simulink model "IKS02A1_VL53L1A1_Both_ROS_fromworkspace_2025b_forstudents"  (R2025b)
settings: Solver=VariableStepAuto  StartTime=0.0  StopTime=out.GT_time.time(end)  RelTol=1e-3
libraries: quarc_library x2
settings Model: Creator=abich  LastModifiedBy=tmood

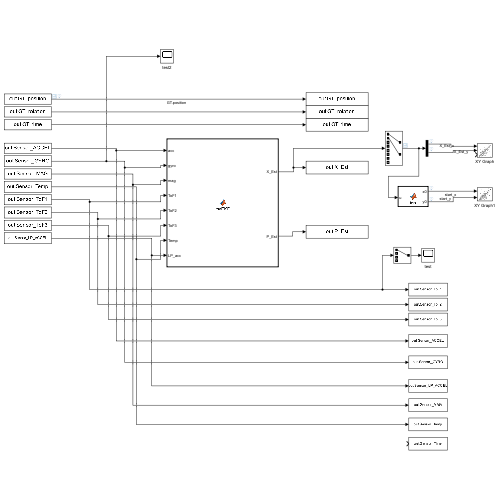
[thumbnail: Simulink's stored preview of the top-level diagram]
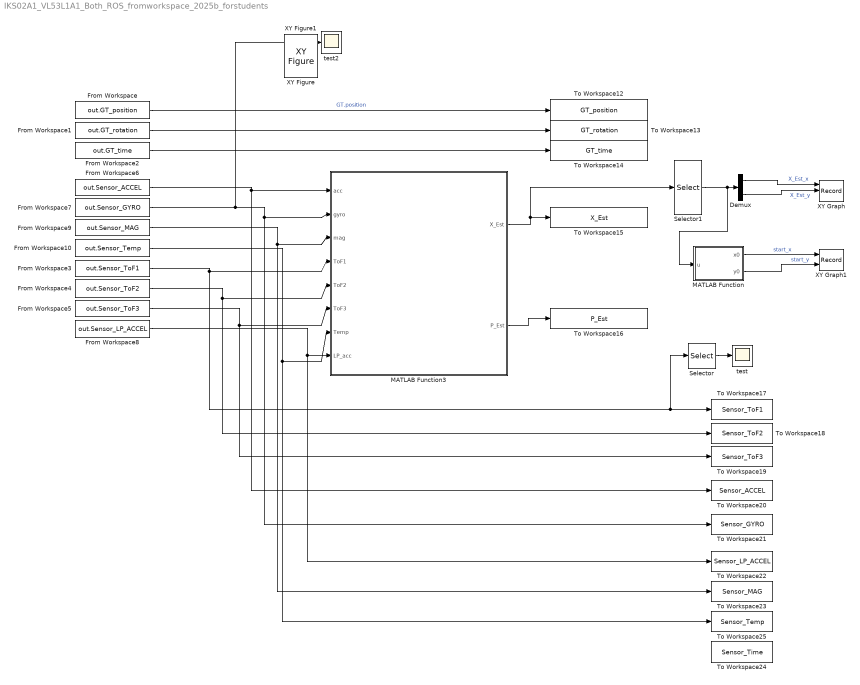
== system IKS02A1_VL53L1A1_Both_ROS_fromworkspace_2025b_forstudents ==
  Demux : Demux  Outputs=2
  From Workspace : FromWorkspace  VariableName=out.GT_position  SampleTime=1/200  OutputAfterFinalValue=Holding final value
  From Workspace1 : FromWorkspace  VariableName=out.GT_rotation  SampleTime=1/200  OutputAfterFinalValue=Holding final value
  From Workspace10 : FromWorkspace  VariableName=out.Sensor_Temp  SampleTime=1/200  OutputAfterFinalValue=Holding final value
  From Workspace2 : FromWorkspace  VariableName=out.GT_time  SampleTime=1/200  OutputAfterFinalValue=Holding final value
  From Workspace3 : FromWorkspace  VariableName=out.Sensor_ToF1  SampleTime=1/200  OutputAfterFinalValue=Holding final value
  From Workspace4 : FromWorkspace  VariableName=out.Sensor_ToF2  SampleTime=1/200  OutputAfterFinalValue=Holding final value
  From Workspace5 : FromWorkspace  VariableName=out.Sensor_ToF3  SampleTime=1/200  OutputAfterFinalValue=Holding final value
  From Workspace6 : FromWorkspace  VariableName=out.Sensor_ACCEL  SampleTime=1/200  OutputAfterFinalValue=Holding final value
  From Workspace7 : FromWorkspace  VariableName=out.Sensor_GYRO  SampleTime=1/200  OutputAfterFinalValue=Holding final value
  From Workspace8 : FromWorkspace  VariableName=out.Sensor_LP_ACCEL  SampleTime=1/200  OutputAfterFinalValue=Holding final value
  From Workspace9 : FromWorkspace  VariableName=out.Sensor_MAG  SampleTime=1/200  OutputAfterFinalValue=Holding final value
  MATLAB Function : MATLAB Function  TreatAsAtomicUnit=on
  MATLAB Function3 : MATLAB Function  TreatAsAtomicUnit=on
  Selector : Selector  InputPortWidth=4  IndexOptions=Index vector (dialog)  Indices=[1]  OutputSizes=1
  Selector1 : Selector  InputPortWidth=8  IndexOptions=Index vector (dialog)  Indices=[1 2]  OutputSizes=1
  To Workspace12 : ToWorkspace  VariableName=GT_position  SaveFormat=Structure With Time  SampleTime=1/200
  To Workspace13 : ToWorkspace  VariableName=GT_rotation  SaveFormat=Structure With Time  SampleTime=1/200
  To Workspace14 : ToWorkspace  VariableName=GT_time  SaveFormat=Structure With Time  SampleTime=1/200
  To Workspace15 : ToWorkspace  VariableName=X_Est  SaveFormat=Structure With Time  SampleTime=1/200
  To Workspace16 : ToWorkspace  VariableName=P_Est  SaveFormat=Structure With Time  SampleTime=1/200
  To Workspace17 : ToWorkspace  VariableName=Sensor_ToF1  SaveFormat=Structure With Time  SampleTime=1/200
  To Workspace18 : ToWorkspace  VariableName=Sensor_ToF2  SaveFormat=Structure With Time  SampleTime=1/200
  To Workspace19 : ToWorkspace  VariableName=Sensor_ToF3  SaveFormat=Structure With Time  SampleTime=1/200
  To Workspace20 : ToWorkspace  VariableName=Sensor_ACCEL  SaveFormat=Structure With Time  SampleTime=1/200
  To Workspace21 : ToWorkspace  VariableName=Sensor_GYRO  SaveFormat=Structure With Time  SampleTime=1/200
  To Workspace22 : ToWorkspace  VariableName=Sensor_LP_ACCEL  SaveFormat=Structure With Time  SampleTime=1/200
  To Workspace23 : ToWorkspace  VariableName=Sensor_MAG  SaveFormat=Structure With Time  SampleTime=1/200
  To Workspace24 : ToWorkspace  VariableName=Sensor_Time  SaveFormat=Structure With Time  SampleTime=1/200
  To Workspace25 : ToWorkspace  VariableName=Sensor_Temp  SaveFormat=Structure With Time  SampleTime=1/200
  XY Graph : Record  NumPorts=3.0  FileSettingsInternal="{\"entries\":[{\"content\":{\"excelSettings\":{\"content\":{},\"type\":\"Streamout.ExcelSettings\"},\"parquetSettings\":{\"content\":{},\"type\":\"Streamout.ParquetSettings\"}},\"type\":\"Streamout.FileSettingStorage\",\"uuid\":\"\"}],\"packageUris\":[\"http:\\/\\/schema.mathworks.com\\/mf0\\/streamout_blocks\\/R2020a\"],\"version\":\"1.0\"}"  FrameSettings=[0, 0, 0]  Layout=[1 1]  SignalsInternal="{\"entries\":[{\"content\":{\"signals\":[{\"content\":{\"blockPath\":[],\"dimensions\":[1],\"domain\":\"\",\"lineColor\":\"#a2142f\",\"plots\":[ 1 ],\"port\":1,\"sid\":[\"\"],\"signalID\":1,\"signalName\":\"X_Est_x\"},\"type\":\"RecordBlkView.Signal\",\"uuid\":\"\"},{\"content\":{\"blockPath\":[],\"dimensions\":[1],\"domain\":\"\",\"lineColor\":\"#139fff\",\"plots\":[ 1 ],\"port\":2,\"sid\":[\"\"],\"signalID\":2,\"signalName\":\"X_Est_y\"},\"type\":\"RecordBlkView.Signal\",\"uuid\":\"\"},{\"content\":{\"blockPath\":[],\"dimensions\":[1],\"domain\":\"\",\"lineColor\":\"#139fff\",\"lineWidth\":2,\"port\":3,\"sid\":[\"\"],\"signalID\":3},\"type\":\"RecordBlkView.Signal\",\"uuid\":\"\"}]},\"type\":\"RecordBlkView.InputSignals\",\"uuid\":\"\"}],\"packageUris\":[\"http:\\/\\/schema.mathworks.com\\/mf0\\/streamout_blocks\\/R2020a\"],\"version\":\"1.0\"}"  VisualizationBindings="{\"xyplotplugin\":{\"info\":[{\"series\":[{\"bindingParametersList\":[{\"parameter\":\"X-Axis\",\"signalID\":1,\"signalName\":\"X_Est_x\"},{\"parameter\":\"Y-Axis\",\"signalID\":2,\"signalName\":\"X_Est_y\"}],\"seriesID\":0}],\"subplotID\":1}]}}"  CompatibilityTag=XY
  XY Graph1 : Record  NumPorts=2.0  FileSettingsInternal="{\"entries\":[{\"content\":{\"excelSettings\":{\"content\":{},\"type\":\"Streamout.ExcelSettings\"},\"parquetSettings\":{\"content\":{},\"type\":\"Streamout.ParquetSettings\"}},\"type\":\"Streamout.FileSettingStorage\",\"uuid\":\"\"}],\"packageUris\":[\"http:\\/\\/schema.mathworks.com\\/mf0\\/streamout_blocks\\/R2020a\"],\"version\":\"1.0\"}"  FrameSettings=[0, 0]  Layout=[1 1]  SignalsInternal="{\"entries\":[{\"content\":{\"signals\":[{\"content\":{\"blockPath\":[],\"dimensions\":[1],\"domain\":\"\",\"lineColor\":\"#a2142f\",\"plots\":[ 1 ],\"port\":1,\"sid\":[\"\"],\"signalID\":1,\"signalName\":\"start_x\"},\"type\":\"RecordBlkView.Signal\",\"uuid\":\"\"},{\"content\":{\"blockPath\":[],\"dimensions\":[1],\"domain\":\"\",\"lineColor\":\"#139fff\",\"plots\":[ 1 ],\"port\":2,\"sid\":[\"\"],\"signalID\":2,\"signalName\":\"start_y\"},\"type\":\"RecordBlkView.Signal\",\"uuid\":\"\"}]},\"type\":\"RecordBlkView.InputSignals\",\"uuid\":\"\"}],\"packageUris\":[\"http:\\/\\/schema.mathworks.com\\/mf0\\/streamout_blocks\\/R2020a\"],\"version\":\"1.0\"}"  VisualizationBindings="{\"xyplotplugin\":{\"info\":[{\"series\":[{\"bindingParametersList\":[{\"parameter\":\"X-Axis\",\"signalID\":1,\"signalName\":\"start_x\"},{\"parameter\":\"Y-Axis\",\"signalID\":2,\"signalName\":\"start_y\"}],\"seriesID\":0}],\"subplotID\":1}]}}"  CompatibilityTag=XY
  test : Scope
      settings: ActiveDisplayYMinimum=-1  ActiveDisplayYMaximum=1
  test2 : Scope
      settings: ActiveDisplayYMinimum=-0.15108420974985681  ActiveDisplayYMaximum=0.16772460685752888  DataLoggingVariableName=ScopeData2
  XY Figure : quarc_library/Sinks/Figures/XY Figure  IOType=viewer  figure_mode=Use figure window  figure_tag=figure1  axes_tag=axes1  plot_mode=Time-based  minimum_x=-1  maximum_x=1  minimum_y=-1  maximum_y=1  buffer_size=1000  update_rate=100  initial_position=[]  initial_visibility=off  sample_time=-1
      settings: SourceProductName=QUARC Targets
  XY Figure1 : quarc_library/Sinks/Figures/XY Figure  IOType=viewer  figure_mode=Use figure window  figure_tag=figure1  axes_tag=axes1  plot_mode=Time-based  minimum_x=-1  maximum_x=1  minimum_y=-1  maximum_y=1  buffer_size=1000  update_rate=100  initial_position=[]  initial_visibility=off  sample_time=-1
      settings: SourceProductName=QUARC Targets
  wires:
  From Workspace4/1 -> To Workspace18/1, MATLAB Function3/5(ToF2)
  From Workspace6/1 -> To Workspace20/1, MATLAB Function3/1(acc)
  From Workspace9/1 -> To Workspace23/1, MATLAB Function3/3(mag)
  From Workspace10/1 -> To Workspace25/1, MATLAB Function3/7(Temp)
  From Workspace2/1 -> To Workspace14/1
  From Workspace5/1 -> To Workspace19/1, MATLAB Function3/6(ToF3)
  MATLAB Function3/1(X_Est) -> Selector1/1, To Workspace15/1
  From Workspace8/1 -> MATLAB Function3/8(LP_acc), To Workspace22/1
  From Workspace3/1 -> Selector/1, To Workspace17/1, MATLAB Function3/4(ToF1)
  From Workspace1/1 -> To Workspace13/1
  From Workspace7/1 -> test2/1, To Workspace21/1, MATLAB Function3/2(gyro)
  MATLAB Function3/2(P_Est) -> To Workspace16/1
  Selector/1 -> test/1
  Selector1/1 -> MATLAB Function/1(u), Demux/1
  Demux/1 -> XY Graph/1  "X_Est_x"
  Demux/2 -> XY Graph/2  "X_Est_y"
  From Workspace/1 -> To Workspace12/1  "GT.position"
  MATLAB Function/1(x0) -> XY Graph1/1  "start_x"
  MATLAB Function/2(y0) -> XY Graph1/2  "start_y"

== matlab function IKS02A1_VL53L1A1_Both_ROS_fromworkspace_2025b_forstudents/MATLAB Function ==
  data: u input; x0 output; y0 output
function [x0,y0] = fcn(u)

x0 = u(1,1);
y0 = u(2,1);
end

== matlab function IKS02A1_VL53L1A1_Both_ROS_fromworkspace_2025b_forstudents/MATLAB Function3 ==
  data: acc input; X_Est output size=8; gyro input; mag input; ToF1 input; ToF2 input; ToF3 input; P_Est output size=[5 5]; Temp input; LP_acc input
function [X_Est, P_Est] = myEKF(acc, gyro, mag, ToF1, ToF2, ToF3, Temp, LP_acc)
% EKF for Sub-Terranean Navigation — Simulink MATLAB Function Block
% Called once per timestep (200Hz, dt=0.005s)
% Inputs (per timestep):
%   acc    : 3x1 accelerometer [ax; ay; az] m/s²
%   gyro   : 3x1 gyroscope     [gx; gy; gz] rad/s  (gx = yaw axis)
%   mag    : 3x1 magnetometer  [mx; my; mz] Tesla
%   ToF1   : 4x1 [dist; ?; ?; status]  left-facing   (alpha=+pi/2)    % *** CHANGED: was right
%   ToF2   : 4x1 [dist; ?; ?; status]  back-facing   (alpha=pi)       % *** CHANGED: was forward
%   ToF3   : 4x1 [dist; ?; ?; status]  right-facing  (alpha=-pi/2)    % *** CHANGED: was left
%   Temp   : unused (template placeholder)
%   LP_acc : unused (template placeholder)
% Outputs:
%   X_Est  : 1x5 [x, y, theta, vx_world, vy_world]
%   P_Est  : 5x5 covariance (top-left block)

%% Persistent state — survives between Simulink timestep calls
persistent X P initialized call_count

% Calibration (computed during startup)
persistent gyro_bias accel_bias_fwd accel_bias_lat
persistent x0 y0 mag_global_offset
persistent ab_xmax ab_xmin ab_ymax ab_ymin

% Mag anomaly detection
persistent theta_gyro_ref gyro_ref_bias mag_disable_until
persistent mag_innov_buf mag_innov_count
persistent gyro_mag_diverge_count prev_innovation_mag mag_innov_growing_count

% ToF rate tracking
persistent prev_tof1_dist prev_tof1_genuine_time
persistent prev_tof2_dist prev_tof2_genuine_time
persistent prev_tof3_dist prev_tof3_genuine_time

% Startup accumulation buffers
persistent startup_gyro startup_accel startup_tof1 startup_tof2 startup_tof3
persistent startup_mag startup_done startup_buf_count

persistent zupt_accel_fwd_buf zupt_accel_lat_buf zupt_gyro_buf zupt_buf_count

%% Constants
dt              = 0.005;

% *** CHANGED: Corrected ToF mounting angles (confirmed by diagnostic) ***
alpha_tof1      =  pi/2;   % was -pi/2 — ToF1 = left
alpha_tof2      =  pi;     % was  0    — ToF2 = back
alpha_tof3      = -pi/2;   % was  pi/2 — ToF3 = right

mag_hard_iron   = [-3.705e-05,  4.415e-05];
mag_soft_iron   = [ 1.0958,     0.9196   ];
theta0          = pi/2;
R_mag           = 4.0;
R_tof           = 0.01;
gamma_threshold = 9.0;

%% First call: initialise all persistent variables
if isempty(initialized)
    call_count   = 0;
    startup_done = false;
    startup_buf_count = 0;

    % Startup buffers — pre-allocate for up to 500 samples
    startup_gyro  = zeros(500, 3);
    startup_accel = zeros(500, 3);
    startup_tof1  = zeros(500, 4);
    startup_tof2  = zeros(500, 4);
    startup_tof3  = zeros(500, 4);
    startup_mag   = zeros(500, 3);

    % Fallback calibration constants (used if startup fails)
    gyro_bias      =  0.00186;
    accel_bias_fwd = -0.396;
    accel_bias_lat =  0.07485;
    x0             =  0.0;
    y0             = -0.93;

    % ZUPT
    zupt_accel_fwd_buf = zeros(40, 1);
    zupt_accel_lat_buf = zeros(40, 1);
    zupt_gyro_buf      = zeros(40, 1);
    zupt_buf_count     = 0;

    % arena_bounds = struct('x_max',  1.22, 'x_min', -1.22, ...
    %                       'y_max',  1.22, 'y_min', -1.22);
    ab_xmax =  1.22; ab_xmin = -1.22;
    ab_ymax =  1.22; ab_ymin = -1.22;

    % These will be properly set after startup completes
    mag_global_offset       = 0;
    theta_gyro_ref          = theta0;
    gyro_ref_bias           = gyro_bias;
    mag_disable_until       = 0;
    mag_innov_buf           = zeros(20, 1);
    mag_innov_count         = 0;
    gyro_mag_diverge_count  = 0;
    prev_innovation_mag     = 0;
    mag_innov_growing_count = 0;

    prev_tof1_dist         = NaN;
    prev_tof1_genuine_time = NaN;
    prev_tof2_dist         = NaN;
    prev_tof2_genuine_time = NaN;
    prev_tof3_dist         = NaN;
    prev_tof3_genuine_time = NaN;

    % State and covariance — will be reset after startup
    X = [0; -0.93; theta0; 0; 0; gyro_bias];
    P = diag([0.1, 0.1, 0.1, 2.0, 2.0, 0.25]);

    initialized = true;
end

call_count = call_count + 1;
current_time = (call_count - 1) * dt;

%% Startup phase: accumulate samples, compute calibration
if ~startup_done
    startup_buf_count = startup_buf_count + 1;
    n = min(startup_buf_count, 500);
    startup_gyro(n, :)  = reshape(gyro,  1, 3);
    startup_accel(n, :) = reshape(acc,   1, 3);
    startup_mag(n, :)   = reshape(mag,   1, 3);
    startup_tof1(n, :)  = reshape(ToF1,  1, 4);
    startup_tof2(n, :)  = reshape(ToF2,  1, 4);
    startup_tof3(n, :)  = reshape(ToF3,  1, 4);

    % *** CHANGED: Use variance-based stationarity detection instead of ***
    % *** absolute threshold. The gyro has a large bias (~-0.49 rad/s)  ***
    % *** so abs(gyro(1)) < 0.01 never triggers. Instead, check if the ***
    % *** gyro reading is STABLE (low variance) over a window.          ***
    if startup_buf_count >= 100
        stat_start   = 0;
        search_limit = min(startup_buf_count, 500);

        % Look for a window of 100 samples where gyro variance is low
        % (robot stationary = constant gyro reading = low variance)
        for i = 100:search_limit
            window = startup_gyro((i-99):i, 1);
            win_var = var(window);
            if win_var < 1e-4   % Low variance = stationary, regardless of bias value
                stat_start = i - 99;
                break;
            end
        end

        if stat_start > 0
            n_stat     = min(200, search_limit - stat_start + 1);
            stat_range = stat_start : (stat_start + n_stat - 1);

            % Per-run calibration
            gyro_bias      = mean(startup_gyro(stat_range, 1));
            accel_bias_fwd = mean(startup_accel(stat_range, 3));
            accel_bias_lat = mean(startup_accel(stat_range, 2));

            % Arena wall + x0/y0 estimation from ToF
            tof1_in = startup_tof1(stat_range, 1);
            tof2_in = startup_tof2(stat_range, 1);
            tof3_in = startup_tof3(stat_range, 1);

            gen1 = tof1_in([true; diff(tof1_in) ~= 0]);
            gen2 = tof2_in([true; diff(tof2_in) ~= 0]);
            gen3 = tof3_in([true; diff(tof3_in) ~= 0]);
            gen1 = gen1(gen1 > 0);
            gen2 = gen2(gen2 > 0);
            gen3 = gen3(gen3 > 0);

            if ~isempty(gen1) && ~isempty(gen2) && ~isempty(gen3)
                s1 = sort(gen1); d_lft = s1(max(1,floor(end/2)));  % *** CHANGED: ToF1=left (was d_rgt)
                s2 = sort(gen2); d_bck = s2(max(1,floor(end/2)));  % *** CHANGED: ToF2=back (was d_fwd)
                s3 = sort(gen3); d_rgt = s3(max(1,floor(end/2)));  % *** CHANGED: ToF3=right (was d_lft)

                if d_lft > 0 && d_bck > 0 && d_rgt > 0 && ...
                   ~isnan(d_lft) && ~isnan(d_bck) && ~isnan(d_rgt)

                    % *** CHANGED: Position estimation using correct ToF mapping ***
                    % At theta0=pi/2: left(+pi/2)=back(+Y), back(pi)=right(+X), right(-pi/2)=forward(-Y)
                    % Actually at theta=pi/2:
                    %   ToF1 left  (+pi/2 from heading): ray = pi/2+pi/2 = pi   → points -X direction → measures dist to -X wall
                    %   ToF2 back  (pi from heading):    ray = pi/2+pi = 3pi/2  → points -Y direction → measures dist to -Y wall
                    %   ToF3 right (-pi/2 from heading): ray = pi/2-pi/2 = 0    → points +X direction → measures dist to +X wall
                    wall_x_max =  1.22;
                    wall_y_max =  1.22;
                    wall_x_min = -1.22;
                    wall_y_min = -1.22;

                    x0 = wall_x_max - d_rgt;     % d_rgt = dist to +X wall
                    y0 = wall_y_min + d_bck;      % d_bck = dist to -Y wall (behind at theta=pi/2 means -Y)

                    % Verify with left sensor: x0 should be close to wall_x_min + d_lft
                    % x0_check = wall_x_min + d_lft;

                    ab_xmax = wall_x_max;
                    ab_xmin = wall_x_min;
                    ab_ymax = wall_y_max;
                    ab_ymin = wall_y_min;
                end
            end

            % Magnetometer global offset
            % *** CHANGED: Use first valid (non-zero) mag sample ***
            mag_init_idx = 1;
            for mi = 1:min(startup_buf_count, 500)
                if norm(startup_mag(mi,:)) > 1e-8
                    mag_init_idx = mi;
                    break;
                end
            end
            mag_y_cal0        = (startup_mag(mag_init_idx,2) - mag_hard_iron(1)) * mag_soft_iron(1);
            mag_z_cal0        = (startup_mag(mag_init_idx,3) - mag_hard_iron(2)) * mag_soft_iron(2);
            z_mag0            = atan2(mag_z_cal0, mag_y_cal0);
            mag_global_offset = wrapToPi_fn(theta0 - z_mag0);

            % Initialise filter state with estimated x0, y0
            X = [x0; y0; theta0; 0; 0; gyro_bias];
            P = diag([0.1, 0.1, 0.1, 2.0, 2.0, 0.25]);

            theta_gyro_ref = theta0;
            gyro_ref_bias  = gyro_bias;

            startup_done = true;
        end
    end

    % During startup, return zero estimates
    X_Est = [0; -0.93; pi/2; 0; 0; 0; 0; 0];   % 1x8
    P_Est = zeros(5, 5);
    return;
end

%% Extract current sensor values
gx      = gyro(1);          % yaw axis gyro (rad/s)
ax_body_raw = acc(3);       % forward accel (m/s²)
ay_body_raw = acc(2);       % lateral accel (m/s²)

tof1_dist   = ToF1(1);
tof1_status = ToF1(4);
tof2_dist   = ToF2(1);
tof2_status = ToF2(4);
tof3_dist   = ToF3(1);
tof3_status = ToF3(4);

mag_y = mag(2);
mag_z = mag(3);

%% Prediction step
omega   = gx - X(6);
Q_base  = diag([1e-4, 1e-4, 1.1e-3, 0.5, 0.5, 1.5e-5]) * dt;

% *** CHANGED: Increased accel clamp from 2.0 to 3.0 — but accel is very ***
% *** noisy (spikes to ±15 m/s²). Consider reducing further or scaling.  ***
ax_body = max(-3.0, min(3.0, ax_body_raw - accel_bias_fwd));
ay_body = max(-3.0, min(3.0, ay_body_raw - accel_bias_lat));

ax_world = ax_body * cos(X(3)) - ay_body * sin(X(3));
ay_world = ax_body * sin(X(3)) + ay_body * cos(X(3));

vel_damp  = 1.0 - 0.5 * dt;

X_pred    = zeros(6, 1);
X_pred(1) = X(1) + X(4) * dt;
X_pred(2) = X(2) + X(5) * dt;
X_pred(3) = wrapToPi_fn(X(3) + omega * dt);
X_pred(4) = X(4) * vel_damp + ax_world * dt;
X_pred(5) = X(5) * vel_damp + ay_world * dt;
X_pred(6) = X(6);

F       = eye(6);
F(1, 4) = dt;
F(2, 5) = dt;
F(3, 6) = -dt;
F(4, 3) = (-ax_body * sin(X(3)) - ay_body * cos(X(3))) * dt;
F(5, 3) = ( ax_body * cos(X(3)) - ay_body * sin(X(3))) * dt;
F(4, 4) = vel_damp;
F(5, 5) = vel_damp;

% Adaptive Q
Q_k = Q_base;
if abs(omega) > 0.15
    Q_k(3,3) = Q_k(3,3) * (1.0 + 9.0 * (abs(omega) - 0.15));
end
if call_count <= mag_disable_until
    Q_k(4,4) = Q_k(4,4) * 1.5;
    Q_k(5,5) = Q_k(5,5) * 1.5;
end
speed = sqrt(X(4)^2 + X(5)^2);
if speed > 0.05
    Q_k(6,6) = Q_k(6,6) * (1.0 + 5.0 * speed);
end

P_pred = F * P * F' + Q_k;
X      = X_pred;
P      = P_pred;

%% Gyro reference update
theta_gyro_ref = wrapToPi_fn(theta_gyro_ref + (gx - gyro_ref_bias) * dt);

%% Magnetometer update with anomaly detection
mag_y_cal = (mag_y - mag_hard_iron(1)) * mag_soft_iron(1);
mag_z_cal = (mag_z - mag_hard_iron(2)) * mag_soft_iron(2);
z_mag     = wrapToPi_fn(atan2(mag_z_cal, mag_y_cal) + mag_global_offset);

innovation_mag = wrapToPi_fn(z_mag - X(3));

% Criterion 1: innovation buffer
mag_innov_count        = mag_innov_count + 1;
buf_idx                = mod(mag_innov_count - 1, 20) + 1;
mag_innov_buf(buf_idx) = innovation_mag;
if mag_innov_count >= 20
    ib_mean   = sum(mag_innov_buf) / 20;
    innov_var = sum((mag_innov_buf - ib_mean).^2) / 19;
    innov_rms = sqrt(sum(mag_innov_buf.^2) / 20);
    if innov_var > 0.04 || innov_rms > 0.15
        mag_disable_until = call_count + 400;
    end
end

% Criterion 2: innovation growing for 5 consecutive steps
if abs(innovation_mag) > abs(prev_innovation_mag) + 0.02
    mag_innov_growing_count = mag_innov_growing_count + 1;
    if mag_innov_growing_count >= 5
        mag_disable_until       = call_count + 400;
        mag_innov_growing_count = 0;
    end
else
    mag_innov_growing_count = max(0, mag_innov_growing_count - 1);
end
prev_innovation_mag = innovation_mag;

% Criterion 3: sustained divergence from gyro reference
gyro_mag_diff = abs(wrapToPi_fn(z_mag - theta_gyro_ref));
max_expected  = 0.008 * current_time + 0.12;
if gyro_mag_diff > max_expected
    gyro_mag_diverge_count = gyro_mag_diverge_count + 1;
    if gyro_mag_diverge_count >= 50
        mag_disable_until      = call_count + 400;
        gyro_mag_diverge_count = 0;
    end
else
    gyro_mag_diverge_count = max(0, gyro_mag_diverge_count - 1);
end

% Apply mag update only when not disabled
if call_count > mag_disable_until
    R_mag_k = 4.0;
    H_mag = [0 0 1 0 0 0];
    S_mag = H_mag * P * H_mag' + R_mag_k;
    if innovation_mag^2 / S_mag < gamma_threshold
        K_mag = P * H_mag' / S_mag;
        X     = X + K_mag * innovation_mag;
        X(3)  = wrapToPi_fn(X(3));
        IKH   = eye(6) - K_mag * H_mag;
        P     = IKH * P * IKH' + K_mag * R_mag_k * K_mag';
        gyro_ref_bias = 0.95 * gyro_ref_bias + 0.05 * X(6);
    end
end

%% ToF distance + rate updates
% ToF 1
if tof1_status == 0
    [h_x, H_tof] = calc_tof(X, ab_xmax, ab_xmin, ab_ymax, ab_ymin, alpha_tof1);
    S          = H_tof * P * H_tof' + R_tof;
    innovation = tof1_dist - h_x;
    if (innovation^2) / S < gamma_threshold
        K    = P * H_tof' / S;
        X    = X + K * innovation;
        X(3) = wrapToPi_fn(X(3));
        IKH  = eye(6) - K * H_tof;
        P    = IKH * P * IKH' + K * R_tof * K';
    end
    tof1_is_new = isnan(prev_tof1_dist) || (tof1_dist ~= prev_tof1_dist);
    if tof1_is_new && ~isnan(prev_tof1_dist) && call_count <= mag_disable_until
        dt_gen = current_time - prev_tof1_genuine_time;
        if dt_gen > 0.08
            spd = sqrt(X(4)^2 + X(5)^2);
            if spd > 0.05 && abs(omega) < 0.2
                phi        = wrapToPi_fn(X(3) + alpha_tof1);
                dro        = (tof1_dist - prev_tof1_dist) / dt_gen;
                dre        = -(X(4)*cos(phi) + X(5)*sin(phi));
                Hr         = zeros(1,6);
                Hr(3)      = X(4)*sin(phi) - X(5)*cos(phi);
                Hr(4)      = -cos(phi);
                Hr(5)      = -sin(phi);
                Sr         = Hr * P * Hr' + 0.5;
                ir         = dro - dre;
                if ir^2 < 9.0 * Sr
                    Kr   = P * Hr' / Sr;
                    X    = X + Kr * ir;
                    X(3) = wrapToPi_fn(X(3));
                    P    = (eye(6) - Kr * Hr) * P;
                end
            end
        end
    end
    if tof1_is_new
        prev_tof1_dist         = tof1_dist;
        prev_tof1_genuine_time = current_time;
    end
end

% ToF 2
if tof2_status == 0
    [h_x, H_tof] = calc_tof(X, ab_xmax, ab_xmin, ab_ymax, ab_ymin, alpha_tof2);
    S          = H_tof * P * H_tof' + R_tof;
    innovation = tof2_dist - h_x;
    if (innovation^2) / S < gamma_threshold
        K    = P * H_tof' / S;
        X    = X + K * innovation;
        X(3) = wrapToPi_fn(X(3));
        IKH  = eye(6) - K * H_tof;
        P    = IKH * P * IKH' + K * R_tof * K';
    end
    tof2_is_new = isnan(prev_tof2_dist) || (tof2_dist ~= prev_tof2_dist);
    if tof2_is_new && ~isnan(prev_tof2_dist) && call_count <= mag_disable_until
        dt_gen = current_time - prev_tof2_genuine_time;
        if dt_gen > 0.08
            spd = sqrt(X(4)^2 + X(5)^2);
            if spd > 0.05 && abs(omega) < 0.2
                phi        = wrapToPi_fn(X(3) + alpha_tof2);
                dro        = (tof2_dist - prev_tof2_dist) / dt_gen;
                dre        = -(X(4)*cos(phi) + X(5)*sin(phi));
                Hr         = zeros(1,6);
                Hr(3)      = X(4)*sin(phi) - X(5)*cos(phi);
                Hr(4)      = -cos(phi);
                Hr(5)      = -sin(phi);
                Sr         = Hr * P * Hr' + 0.5;
                ir         = dro - dre;
                if ir^2 < 9.0 * Sr
                    Kr   = P * Hr' / Sr;
                    X    = X + Kr * ir;
                    X(3) = wrapToPi_fn(X(3));
                    P    = (eye(6) - Kr * Hr) * P;
                end
            end
        end
    end
    if tof2_is_new
        prev_tof2_dist         = tof2_dist;
        prev_tof2_genuine_time = current_time;
    end
end

% ToF 3
if tof3_status == 0
    [h_x, H_tof] = calc_tof(X, ab_xmax, ab_xmin, ab_ymax, ab_ymin, alpha_tof3);
    S          = H_tof * P * H_tof' + R_tof;
    innovation = tof3_dist - h_x;
    if (innovation^2) / S < gamma_threshold
        K    = P * H_tof' / S;
        X    = X + K * innovation;
        X(3) = wrapToPi_fn(X(3));
        IKH  = eye(6) - K * H_tof;
        P    = IKH * P * IKH' + K * R_tof * K';
    end
    tof3_is_new = isnan(prev_tof3_dist) || (tof3_dist ~= prev_tof3_dist);
    if tof3_is_new && ~isnan(prev_tof3_dist) && call_count <= mag_disable_until
        dt_gen = current_time - prev_tof3_genuine_time;
        if dt_gen > 0.08
            spd = sqrt(X(4)^2 + X(5)^2);
            if spd > 0.05 && abs(omega) < 0.2
                phi        = wrapToPi_fn(X(3) + alpha_tof3);
                dro        = (tof3_dist - prev_tof3_dist) / dt_gen;
                dre        = -(X(4)*cos(phi) + X(5)*sin(phi));
                Hr         = zeros(1,6);
                Hr(3)      = X(4)*sin(phi) - X(5)*cos(phi);
                Hr(4)      = -cos(phi);
                Hr(5)      = -sin(phi);
                Sr         = Hr * P * Hr' + 0.5;
                ir         = dro - dre;
                if ir^2 < 9.0 * Sr
                    Kr   = P * Hr' / Sr;
                    X    = X + Kr * ir;
                    X(3) = wrapToPi_fn(X(3));
                    P    = (eye(6) - Kr * Hr) * P;
                end
            end
        end
    end
    if tof3_is_new
        prev_tof3_dist         = tof3_dist;
        prev_tof3_genuine_time = current_time;
    end
end

%% ZUPT — 40-sample variance window
zupt_buf_count = zupt_buf_count + 1;
buf_i = mod(zupt_buf_count - 1, 40) + 1;
zupt_accel_fwd_buf(buf_i) = ax_body;
zupt_accel_lat_buf(buf_i) = ay_body;
zupt_gyro_buf(buf_i)      = gx;

if zupt_buf_count >= 40
    az_mean  = sum(zupt_accel_fwd_buf) / 40;
    ay_mean  = sum(zupt_accel_lat_buf) / 40;
    gy_mean  = sum(zupt_gyro_buf) / 40;
    az_var   = sum((zupt_accel_fwd_buf - az_mean).^2) / 39;
    ay_var   = sum((zupt_accel_lat_buf - ay_mean).^2) / 39;
    gyro_var = sum((zupt_gyro_buf - gy_mean).^2) / 39;

    if az_var < 0.005 && ay_var < 0.005 && gyro_var < 0.0005
        % Part 1: Velocity ZUPT
        H_v     = [0 0 0 1 0 0; 0 0 0 0 1 0];
        innov_v = -[X(4); X(5)];
        S_v     = H_v * P * H_v' + 0.002 * eye(2);
        K_v     = P * H_v' / S_v;
        X       = X + K_v * innov_v;
        P       = (eye(6) - K_v * H_v) * P;

        % Part 2: Gyro bias ZUPT
        H_b     = [0 0 0 0 0 1];
        innov_b = gx - X(6);
        S_b     = P(6,6) + 0.00005;
        K_b     = P * H_b' / S_b;
        X       = X + K_b * innov_b;
        P       = (eye(6) - K_b * H_b) * P;
        gyro_ref_bias = X(6);

        % Part 3: Soft heading ZUPT
        H_h     = [0 0 1 0 0 0];
        innov_h = -(omega * dt);
        S_h     = H_h * P * H_h' + 0.005;
        K_h     = P * H_h' / S_h;
        X       = X + K_h * innov_h;
        X(3)    = wrapToPi_fn(X(3));
        P       = (eye(6) - K_h * H_h) * P;
    end
end

%% Output current state estimate
X_Est = [X(1:5); 0; 0; 0];    % 1x8 — padded to match model expectation
P_Est = P(1:5, 1:5);           % 5x5

end  % function myEKF

%% Local helper: ToF measurement model
function [h_x, H_tof] = calc_tof(X, xmax, xmin, ymax, ymin, alpha)
    x   = X(1);
    y   = X(2);
    phi = mod(X(3) + alpha + pi, 2*pi) - pi;

    d_right  = inf; d_left = inf; d_top = inf; d_bottom = inf;

    if cos(phi) > 1e-6
        d_right = (xmax - x) / cos(phi);
    elseif cos(phi) < -1e-6
        d_left  = (xmin - x) / cos(phi);
    end
    if sin(phi) > 1e-6
        d_top    = (ymax - y) / sin(phi);
    elseif sin(phi) < -1e-6
        d_bottom = (ymin - y) / sin(phi);
    end

    distances = [d_right, d_left, d_top, d_bottom];
    distances(distances <= 0) = inf;
    [h_x, wall_idx] = min(distances);

    if isinf(h_x)
        H_tof = zeros(1, length(X));
        return;
    end

    H_tof = zeros(1, 6);
    if wall_idx == 1 || wall_idx == 2
        H_tof(1) = -1 / cos(phi);
        H_tof(3) = 0;
    else
        H_tof(2) = -1 / sin(phi);
        H_tof(3) = 0;
    end
end

%% Local helper: angle wrapping
function a = wrapToPi_fn(a)
    a = mod(a + pi, 2*pi) - pi;
end
